simulink model "Replay_sim"  (Simulink 7.8)
settings: Solver=FixedStepDiscrete  StartTime=0.0  StopTime=valid_range_time(end)  FixedStep=T_step  RelTol=1e-3
InitFcn:
  | Replay_sim_init
values from neighbouring files (symbols this model uses):
  InitialPoint = 0    [boat_constants.m]    (also in l2plus.m)
  IPStar = 0    [boat_constants.m]    (also in l2plus.m)
  lla_ltp_gain = [r * (pi / 180 / 1e7); v * cos(ref_lla(1)) * (pi / 180 / 1e7); 1e-6]    [common.m]
  MaxDwnPthStar = 1    [boat_constants.m]    (also in l2plus.m)
  switchDistance = 4    [boat_constants.m]    (also in l2plus.m)
  T_step = 0.01    [boat_constants.m]    (also in common.m)
  tanIntercept = tan( 45*pi/180 )    [boat_constants.m]    (also in l2plus.m)
  TStar = single(4.5)    [boat_constants.m]    (also in l2plus.m = single(2))
  Turn2Track = 0    [boat_constants.m]    (also in l2plus.m)
  wheelbase = 3.27    [boat_constants.m]
undefined symbols (not defined in the file or in its folder): cogDotDerivativeDelay, DiscIntNeverNeededParam, gpsOrigin, KPsiDot
settings Model: Creator=Bryant  LastModifiedBy=Bryant
settings OptimizationCC: LifeSpan=30

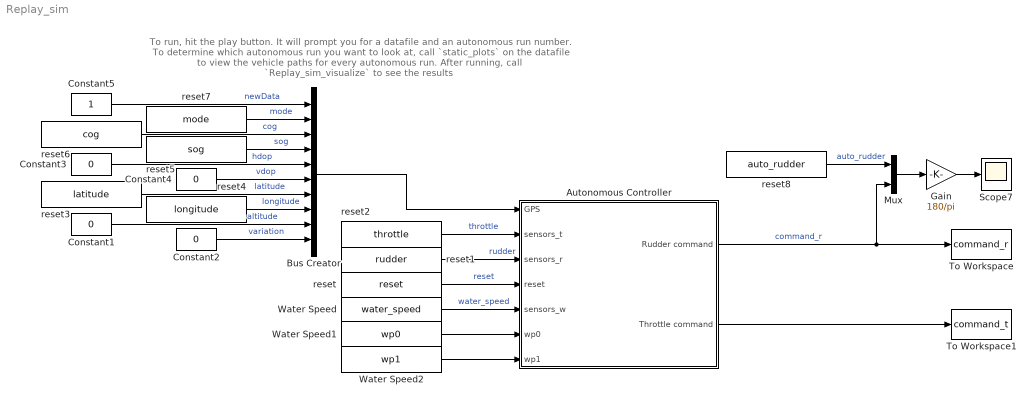
== system Replay_sim ==
  note: To run, hit the play button. It will prompt you for a datafile and an autonomous run number.
      |
      | To determine which autonomous run you want to look at, call `static_plots` on the datafile to
      | view the vehicle paths for every autonomous run.
      |
      | After running, call `Replay_sim_visualize` to see the results
  Autonomous Controller : Subsystem  Priority=1
  Bus Creator : BusCreator  Inputs=10  OutDataTypeStr=Bus: GpsData
  Constant1 : Constant  Value=0  OutDataTypeStr=int32
  Constant2 : Constant  Value=0  OutDataTypeStr=single
  Constant3 : Constant  Value=0  OutDataTypeStr=int16
  Constant4 : Constant  Value=0  OutDataTypeStr=int16
  Constant5 : Constant  OutDataTypeStr=boolean
  Gain : Gain  Gain=180/pi
  Mux : Mux  Inputs=2
  Scope7 : Scope
      settings: SaveName=ScopeData7
  To Workspace : ToWorkspace  VariableName=command_r  SampleTime=-1  SaveFormat=Structure With Time
  To Workspace1 : ToWorkspace  VariableName=command_t  SampleTime=-1  SaveFormat=Structure With Time
  Water Speed : FromWorkspace  VariableName=water_speed  SampleTime=T_step  Interpolate=off  OutputAfterFinalValue=Holding final value
  Water Speed1 : FromWorkspace  VariableName=wp0  SampleTime=T_step  Interpolate=off  OutputAfterFinalValue=Holding final value
  Water Speed2 : FromWorkspace  VariableName=wp1  SampleTime=T_step  Interpolate=off  OutputAfterFinalValue=Holding final value
  reset : FromWorkspace  VariableName=reset  SampleTime=T_step  Interpolate=off  OutputAfterFinalValue=Holding final value
  reset1 : FromWorkspace  VariableName=rudder  SampleTime=T_step  Interpolate=off  OutputAfterFinalValue=Holding final value
  reset2 : FromWorkspace  VariableName=throttle  SampleTime=T_step  Interpolate=off  OutputAfterFinalValue=Holding final value
  reset3 : FromWorkspace  VariableName=latitude  SampleTime=T_step  Interpolate=off  OutputAfterFinalValue=Holding final value
  reset4 : FromWorkspace  VariableName=longitude  SampleTime=T_step  Interpolate=off  OutputAfterFinalValue=Holding final value
  reset5 : FromWorkspace  VariableName=sog  SampleTime=T_step  Interpolate=off  OutputAfterFinalValue=Holding final value
  reset6 : FromWorkspace  VariableName=cog  SampleTime=T_step  Interpolate=off  OutputAfterFinalValue=Holding final value
  reset7 : FromWorkspace  VariableName=mode  SampleTime=T_step  Interpolate=off  OutputAfterFinalValue=Holding final value
  reset8 : FromWorkspace  VariableName=auto_rudder  SampleTime=T_step  Interpolate=off  OutputAfterFinalValue=Holding final value
  wires:
  Water Speed/1 -> Autonomous Controller/5(sensors_w)  "water_speed"
  Autonomous Controller/2(Throttle command) -> To Workspace1/1
  Autonomous Controller/1(Rudder command) -> To Workspace/1, Mux/2  "command_r"
  reset/1 -> Autonomous Controller/4(reset)  "reset"
  reset1/1 -> Autonomous Controller/3(sensors_r)  "rudder"
  reset2/1 -> Autonomous Controller/2(sensors_t)  "throttle"
  reset3/1 -> Bus Creator/7  "latitude"
  Bus Creator/1 -> Autonomous Controller/1(GPS)
  reset4/1 -> Bus Creator/8  "longitude"
  Constant2/1 -> Bus Creator/10  "variation"
  Constant1/1 -> Bus Creator/9  "altitude"
  Constant4/1 -> Bus Creator/6  "vdop"
  Constant3/1 -> Bus Creator/5  "hdop"
  reset5/1 -> Bus Creator/4  "sog"
  reset6/1 -> Bus Creator/3  "cog"
  reset7/1 -> Bus Creator/2  "mode"
  Constant5/1 -> Bus Creator/1  "newData"
  Mux/1 -> Gain/1
  reset8/1 -> Mux/1  "auto_rudder"
  Water Speed2/1 -> Autonomous Controller/7(wp1)
  Water Speed1/1 -> Autonomous Controller/6(wp0)
  Gain/1 -> Scope7/1

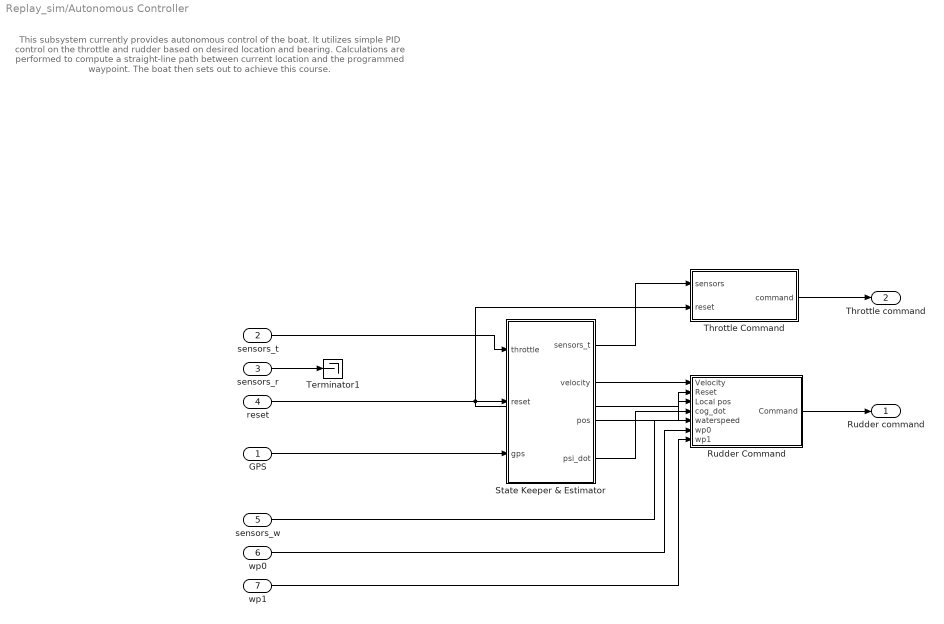
== system Replay_sim/Autonomous Controller ==
  note: This subsystem currently provides autonomous control of the boat. It utilizes simple PID control
      | on the throttle and rudder based on desired location and bearing. Calculations are performed
      | to compute a straight-line path between current location and the programmed waypoint. The
      | boat then sets out to achieve this course.
  GPS : Inport
  sensors_t : Inport  Port=2
  sensors_r : Inport  Port=3
  reset : Inport  Port=4
  sensors_w : Inport  Port=5
  wp0 : Inport  Port=6
  wp1 : Inport  Port=7
  Rudder Command : Subsystem
  State Keeper & Estimator : Subsystem
  Terminator1 : Terminator
  Throttle Command : Subsystem
  Rudder command : Outport
  Throttle command : Outport  Port=2
  wires:
  reset/1 -> Rudder Command/2(Reset), Throttle Command/2(reset), State Keeper & Estimator/2(reset)
  State Keeper & Estimator/3(pos) -> Rudder Command/3(Local pos)
  State Keeper & Estimator/1(sensors_t) -> Throttle Command/1(sensors)
  State Keeper & Estimator/2(velocity) -> Rudder Command/1(Velocity)
  GPS/1 -> State Keeper & Estimator/3(gps)
  Throttle Command/1(command) -> Throttle command/1
  Rudder Command/1(Command) -> Rudder command/1
  sensors_r/1 -> Terminator1/1
  sensors_t/1 -> State Keeper & Estimator/1(throttle)
  State Keeper & Estimator/4(psi_dot) -> Rudder Command/4(cog_dot)
  sensors_w/1 -> Rudder Command/5(waterspeed)
  wp0/1 -> Rudder Command/6(wp0)
  wp1/1 -> Rudder Command/7(wp1)

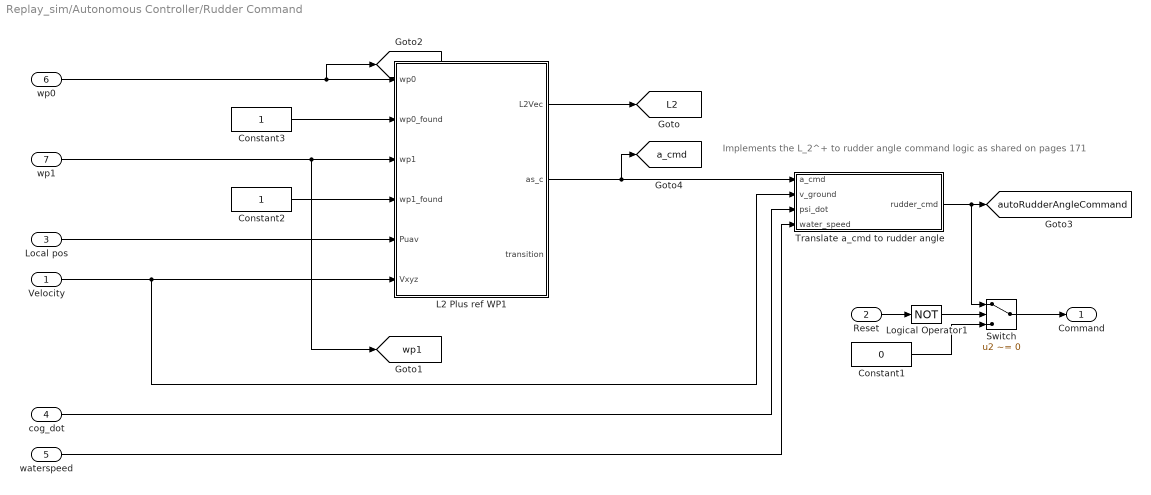
== system Replay_sim/Autonomous Controller/Rudder Command ==
  note: Implements the L_2^+ to rudder angle command logic as shared on pages 171
  Velocity : Inport
  Reset : Inport  Port=2
  Local pos : Inport  Port=3
  cog_dot : Inport  Port=4
  waterspeed : Inport  Port=5
  wp0 : Inport  Port=6
  wp1 : Inport  Port=7
  Constant1 : Constant  Value=0  OutDataTypeStr=single
  Constant2 : Constant  OutDataTypeStr=boolean
  Constant3 : Constant  OutDataTypeStr=boolean
  L2 Plus ref WP1 : MATLAB Function  TreatAsAtomicUnit=on
  Logical Operator1 : Logic  Operator=NOT  Inputs=1  AllPortsSameDT=off  OutDataTypeStr=boolean
  Switch : Switch  Criteria=u2 ~= 0
  Translate a_cmd to rudder angle : Subsystem
  Command : Outport
  tag scope: L2=global, a_cmd=global, autoRudderAngleCommand=global, wp0=global, wp1=global
  wires:
  wp0/1 -> L2 Plus ref WP1/1(wp0), [wp0]
  wp1/1 -> L2 Plus ref WP1/3(wp1), [wp1]
  Local pos/1 -> L2 Plus ref WP1/5(Puav)
  Velocity/1 -> L2 Plus ref WP1/6(Vxyz), Translate a_cmd to rudder angle/2(v_ground)
  L2 Plus ref WP1/1(L2Vec) -> [L2]
  Translate a_cmd to rudder angle/1(rudder_cmd) -> [autoRudderAngleCommand], Switch/1
  Reset/1 -> Logical Operator1/1
  Constant1/1 -> Switch/3
  Switch/1 -> Command/1
  Logical Operator1/1 -> Switch/2
  L2 Plus ref WP1/2(as_c) -> [a_cmd], Translate a_cmd to rudder angle/1(a_cmd)
  cog_dot/1 -> Translate a_cmd to rudder angle/3(psi_dot)
  waterspeed/1 -> Translate a_cmd to rudder angle/4(water_speed)
  Constant3/1 -> L2 Plus ref WP1/2(wp0_found)
  Constant2/1 -> L2 Plus ref WP1/4(wp1_found)

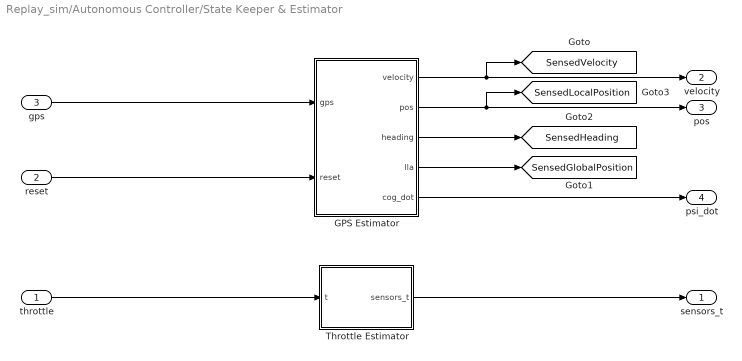
== system Replay_sim/Autonomous Controller/State Keeper & Estimator ==
  throttle : Inport
  reset : Inport  Port=2
  gps : Inport  Port=3
  GPS Estimator : Subsystem
  Throttle Estimator : Subsystem
  sensors_t : Outport
  velocity : Outport  Port=2
  pos : Outport  Port=3
  psi_dot : Outport  Port=4
  tag scope: SensedGlobalPosition=global, SensedHeading=global, SensedLocalPosition=global, SensedVelocity=global
  wires:
  Throttle Estimator/1(sensors_t) -> sensors_t/1
  GPS Estimator/4(lla) -> [SensedGlobalPosition]
  GPS Estimator/3(heading) -> [SensedHeading]
  GPS Estimator/2(pos) -> [SensedLocalPosition], pos/1
  gps/1 -> GPS Estimator/1(gps)
  GPS Estimator/1(velocity) -> [SensedVelocity], velocity/1
  reset/1 -> GPS Estimator/2(reset)
  throttle/1 -> Throttle Estimator/1(t)
  GPS Estimator/5(cog_dot) -> psi_dot/1

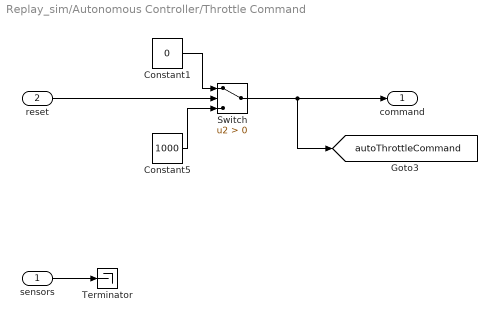
== system Replay_sim/Autonomous Controller/Throttle Command ==
  sensors : Inport
  reset : Inport  Port=2
  Constant1 : Constant  Value=0  OutDataTypeStr=int16
  Constant5 : Constant  Value=1000  OutDataTypeStr=int16
  Switch : Switch  Criteria=u2 > Threshold
  Terminator : Terminator
  command : Outport
  tag scope: autoThrottleCommand=global
  wires:
  Constant5/1 -> Switch/3
  Constant1/1 -> Switch/1
  reset/1 -> Switch/2
  sensors/1 -> Terminator/1
  Switch/1 -> [autoThrottleCommand], command/1

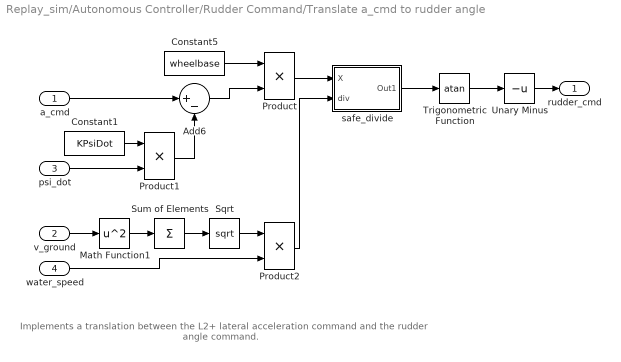
== system Replay_sim/Autonomous Controller/Rudder Command/Translate a_cmd to rudder angle ==
  note: Implements a translation between the L2+ lateral acceleration command
      | and the rudder angle command.
  a_cmd : Inport
  v_ground : Inport  Port=2
  psi_dot : Inport  Port=3
  water_speed : Inport  Port=4
  Add6 : Sum  Inputs=|+-
  Constant1 : Constant  Value=KPsiDot
  Constant5 : Constant  Value=wheelbase
  Math Function1 : Math  Operator=square  SaturateOnIntegerOverflow=on
  Product : Product  Inputs=**  RndMeth=Zero
  Product1 : Product  Inputs=**  RndMeth=Zero
  Product2 : Product  Inputs=**  RndMeth=Zero
  Sqrt : Sqrt  SaturateOnIntegerOverflow=on
  Sum of Elements : Sum  Inputs=+
  Trigonometric Function : Trigonometry  Operator=atan
  Unary Minus : UnaryMinus
  safe_divide : Subsystem  TreatAsAtomicUnit=on
      settings: RTWFcnNameOpts=Use subsystem name  RTWFileNameOpts=Use function name
  rudder_cmd : Outport
  wires:
  Constant5/1 -> Product/1
  Product/1 -> safe_divide/1(X)
  Trigonometric Function/1 -> Unary Minus/1
  Math Function1/1 -> Sum of Elements/1
  Sum of Elements/1 -> Sqrt/1
  safe_divide/1(Out1) -> Trigonometric Function/1
  Add6/1 -> Product/2
  Product1/1 -> Add6/2
  v_ground/1 -> Math Function1/1
  Unary Minus/1 -> rudder_cmd/1
  a_cmd/1 -> Add6/1
  psi_dot/1 -> Product1/2
  Constant1/1 -> Product1/1
  Sqrt/1 -> Product2/1
  Product2/1 -> safe_divide/2(div)
  water_speed/1 -> Product2/2

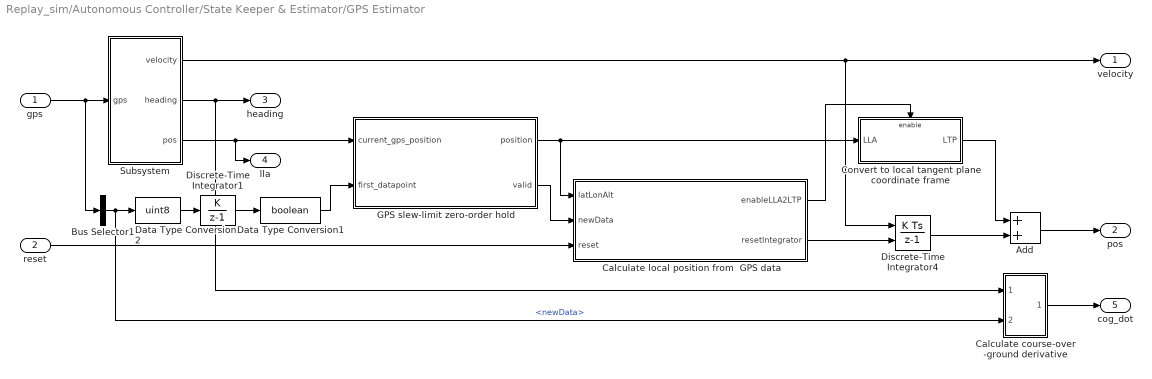
== system Replay_sim/Autonomous Controller/State Keeper & Estimator/GPS Estimator ==
  gps : Inport
  reset : Inport  Port=2
  Add : Sum
  Bus Selector1 : BusSelector  OutputSignals=newData
  Calculate course-over-ground derivative : Subsystem
  Calculate local position from  GPS data : MATLAB Function  TreatAsAtomicUnit=on
  Convert to local tangent plane coordinate frame : Subsystem  TreatAsAtomicUnit=on  RTWFcnName=lla2ltp
      settings: RTWFcnNameOpts=User specified
  Data Type Conversion1 : DataTypeConversion  OutDataTypeStr=boolean
  Data Type Conversion2 : DataTypeConversion  OutDataTypeStr=uint8
  Discrete-Time Integrator1 : DiscreteIntegrator  IntegratorMethod=Accumulation: Forward Euler  SampleTime=-1  OutDataTypeStr=uint8  RndMeth=Simplest  LimitOutput=on  UpperSaturationLimit=1  LowerSaturationLimit=0  ICPrevOutput=DiscIntNeverNeededParam  ICPrevScaledInput=DiscIntNeverNeededParam
  Discrete-Time Integrator4 : DiscreteIntegrator  ExternalReset=level  SampleTime=-1  ICPrevOutput=DiscIntNeverNeededParam  ICPrevScaledInput=DiscIntNeverNeededParam
  GPS slew-limit zero-order hold : MATLAB Function  TreatAsAtomicUnit=on
  Subsystem : Subsystem
  velocity : Outport
  pos : Outport  Port=2
  heading : Outport  Port=3
  lla : Outport  Port=4
  cog_dot : Outport  Port=5
  wires:
  Subsystem/1(velocity) -> Discrete-Time Integrator4/1, velocity/1
  Calculate local position from  GPS data/2(resetIntegrator) -> Discrete-Time Integrator4/2
  Add/1 -> pos/1
  Discrete-Time Integrator4/1 -> Add/2
  Subsystem/3(pos) -> lla/1, GPS slew-limit zero-order hold/1(current_gps_position)
  gps/1 -> Bus Selector1/1, Subsystem/1(gps)
  Subsystem/2(heading) -> heading/1, Calculate course-over-ground derivative/1(cog)
  reset/1 -> Calculate local position from  GPS data/3(reset)
  Convert to local tangent plane coordinate frame/1(LTP) -> Add/1
  Calculate local position from  GPS data/1(enableLLA2LTP) -> Convert to local tangent plane coordinate frame/Enable
  Discrete-Time Integrator1/1 -> Data Type Conversion1/1
  GPS slew-limit zero-order hold/1(position) -> Calculate local position from  GPS data/1(latLonAlt), Convert to local tangent plane coordinate frame/1(LLA)
  GPS slew-limit zero-order hold/2(valid) -> Calculate local position from  GPS data/2(newData)
  Bus Selector1/1 -> Calculate course-over-ground derivative/2(new), Data Type Conversion2/1  "<newData>"
  Data Type Conversion1/1 -> GPS slew-limit zero-order hold/2(first_datapoint)
  Data Type Conversion2/1 -> Discrete-Time Integrator1/1
  Calculate course-over-ground derivative/1(cog_dot) -> cog_dot/1

== system Replay_sim/Autonomous Controller/State Keeper & Estimator/Throttle Estimator ==
  t : Inport
  sensors_t : Outport
  wires:
  t/1 -> sensors_t/1

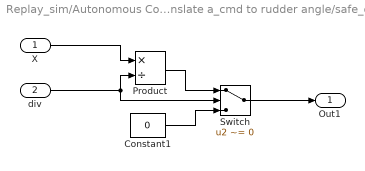
== system Replay_sim/Autonomous Controller/Rudder Command/Translate a_cmd to rudder angle/safe_divide ==
  X : Inport
  div : Inport  Port=2
  Constant1 : Constant  Value=0  OutDataTypeStr=Inherit: Inherit via back propagation
  Product : Product  Inputs=*/  RndMeth=Zero
  Switch : Switch  Criteria=u2 ~= 0
  Out1 : Outport
  wires:
  X/1 -> Product/1
  div/1 -> Product/2, Switch/2
  Product/1 -> Switch/1
  Constant1/1 -> Switch/3
  Switch/1 -> Out1/1

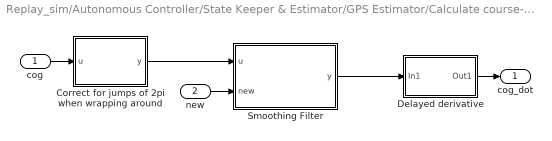
== system Replay_sim/Autonomous Controller/State Keeper & Estimator/GPS Estimator/Calculate course-over-ground derivative ==
  cog : Inport
  new : Inport  Port=2
  Correct for jumps of 2pi when wrapping around : MATLAB Function  TreatAsAtomicUnit=on
  Delayed derivative : Subsystem  mask{delay=cogDotDerivativeDelay, Ts=.01}
      mask prompts: delay "Delay (s)"; Ts "Sample time"
      mask Display: text(0.5,0.5,'Der');
  Smoothing Filter : Subsystem  mask{gain=0.5, limit=8, Ts=.01, freq=.3}
      mask prompts: Ts "Sample time"; freq "Lowpass frequency"
  cog_dot : Outport
  wires:
  Smoothing Filter/1(y) -> Delayed derivative/1(In1)
  Correct for jumps of 2pi when wrapping around/1(y) -> Smoothing Filter/1(u)
  cog/1 -> Correct for jumps of 2pi when wrapping around/1(u)
  Delayed derivative/1(Out1) -> cog_dot/1
  new/1 -> Smoothing Filter/2(new)

== system Replay_sim/Autonomous Controller/State Keeper & Estimator/GPS Estimator/Convert to local tangent plane coordinate frame ==
  LLA : Inport
  Enable : EnablePort
  LLA2LTP : Subsystem  TreatAsAtomicUnit=on  RTWFcnName=lla2ltp
      settings: RTWFcnNameOpts=User specified
  LTP : Outport  OutDataTypeStr=single  InitialOutput=[0, 0, 0]
  wires:
  LLA/1 -> LLA2LTP/1(LLA)
  LLA2LTP/1(LTP) -> LTP/1

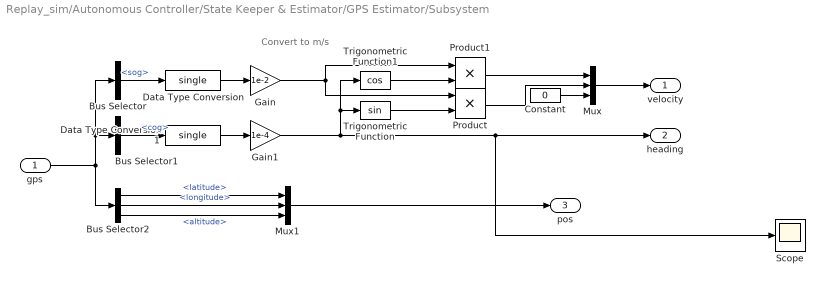
== system Replay_sim/Autonomous Controller/State Keeper & Estimator/GPS Estimator/Subsystem ==
  note: Convert to m/s
  gps : Inport
  Bus Selector : BusSelector  OutputSignals=sog
  Bus Selector1 : BusSelector  OutputSignals=cog
  Bus Selector2 : BusSelector  OutputSignals=latitude,longitude,altitude
  Constant : Constant  Value=0  OutDataTypeStr=single
  Data Type Conversion : DataTypeConversion  OutDataTypeStr=single  RndMeth=Simplest
  Data Type Conversion1 : DataTypeConversion  OutDataTypeStr=single  RndMeth=Simplest
  Gain : Gain  Gain=1e-2
  Gain1 : Gain  Gain=1e-4
  Mux : Mux  Inputs=3
  Mux1 : Mux  Inputs=3
  Product : Product  OutDataTypeStr=single  RndMeth=Zero
  Product1 : Product  OutDataTypeStr=single  RndMeth=Zero
  Scope : Scope
      settings: YMin=1.6  YMax=1.825
  Trigonometric Function : Trigonometry
  Trigonometric Function1 : Trigonometry  Operator=cos
  velocity : Outport
  heading : Outport  Port=2
  pos : Outport  Port=3
  wires:
  gps/1 -> Bus Selector/1, Bus Selector1/1, Bus Selector2/1
  Bus Selector1/1 -> Data Type Conversion1/1  "<cog>"
  Trigonometric Function/1 -> Product/2
  Trigonometric Function1/1 -> Product1/2
  Product1/1 -> Mux/1
  Product/1 -> Mux/2
  Constant/1 -> Mux/3
  Mux/1 -> velocity/1
  Bus Selector/1 -> Data Type Conversion/1  "<sog>"
  Bus Selector2/2 -> Mux1/2  "<longitude>"
  Bus Selector2/3 -> Mux1/3  "<altitude>"
  Mux1/1 -> pos/1
  Bus Selector2/1 -> Mux1/1  "<latitude>"
  Data Type Conversion/1 -> Gain/1
  Data Type Conversion1/1 -> Gain1/1
  Gain/1 -> Product1/1, Product/1
  Gain1/1 -> Trigonometric Function/1, Trigonometric Function1/1, heading/1, Scope/1

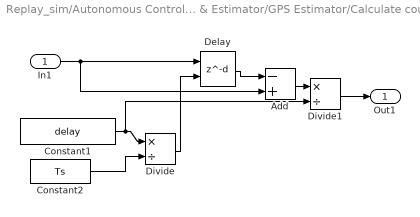
== system Replay_sim/Autonomous Controller/State Keeper & Estimator/GPS Estimator/Calculate course-over-ground derivative/Delayed derivative ==
  In1 : Inport
  Add : Sum  Inputs=-+
  Constant1 : Constant  Value=delay  OutDataTypeStr=single  SampleTime=.01
  Constant2 : Constant  Value=Ts  OutDataTypeStr=single
  Delay : Delay  DelayLengthSource=Input port  DelayLength=delay/Ts  DelayLengthUpperLimit=1000  DiagnosticForOutOfRangeDelayLength=Error  RemoveProtectionDelayLength=on  UseCircularBuffer=on  SampleTime=.01
      settings: InputPortMap=u0,p1
  Divide : Product  Inputs=*/
  Divide1 : Product  Inputs=*/
  Out1 : Outport
  wires:
  Delay/1 -> Add/1
  Add/1 -> Divide1/1
  In1/1 -> Delay/1, Add/2
  Divide1/1 -> Out1/1
  Divide/1 -> Delay/2
  Constant1/1 -> Divide1/2, Divide/1
  Constant2/1 -> Divide/2

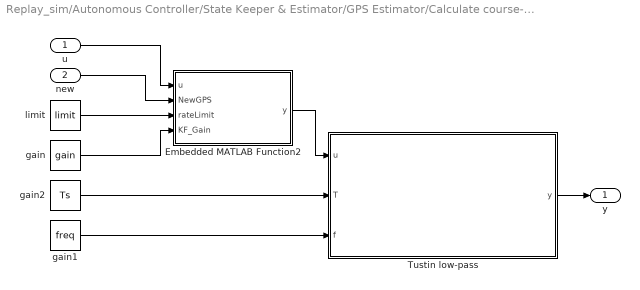
== system Replay_sim/Autonomous Controller/State Keeper & Estimator/GPS Estimator/Calculate course-over-ground derivative/Smoothing Filter ==
  u : Inport  OutDataTypeStr=single
  new : Inport  Port=2  OutDataTypeStr=boolean
  Embedded MATLAB Function2 : MATLAB Function  TreatAsAtomicUnit=on
  Tustin low-pass : MATLAB Function  TreatAsAtomicUnit=on
  gain : Constant  Value=gain  OutDataTypeStr=Inherit: Inherit via back propagation
  gain1 : Constant  Value=freq  OutDataTypeStr=Inherit: Inherit via back propagation
  gain2 : Constant  Value=Ts  OutDataTypeStr=Inherit: Inherit via back propagation
  limit : Constant  Value=limit  OutDataTypeStr=Inherit: Inherit via back propagation
  y : Outport  OutputWhenDisabled=reset  InitialOutput=0
  wires:
  Embedded MATLAB Function2/1(y) -> Tustin low-pass/1(u)
  u/1 -> Embedded MATLAB Function2/1(u)
  new/1 -> Embedded MATLAB Function2/2(NewGPS)
  limit/1 -> Embedded MATLAB Function2/3(rateLimit)
  gain/1 -> Embedded MATLAB Function2/4(KF_Gain)
  Tustin low-pass/1(y) -> y/1
  gain2/1 -> Tustin low-pass/2(T)
  gain1/1 -> Tustin low-pass/3(f)

== system Replay_sim/Autonomous Controller/State Keeper & Estimator/GPS Estimator/Convert to local tangent plane coordinate frame/LLA2LTP ==
  LLA : Inport
  Add : Sum  Inputs=+-  OutDataTypeStr=double  RndMeth=Simplest
  Constant : Constant  Value=gpsOrigin  OutDataTypeStr=int32
  Constant1 : Constant  Value=lla_ltp_gain  OutDataTypeStr=double
  Product : Product  OutDataTypeStr=single  RndMeth=Simplest  LockScale=on
  LTP : Outport  OutDataTypeStr=single  InitialOutput=[0, 0, 0]
  wires:
  Add/1 -> Product/1
  Constant1/1 -> Product/2
  Product/1 -> LTP/1
  Constant/1 -> Add/2
  LLA/1 -> Add/1

== matlab function Autonomous Controller/State Keeper & Estimator/GPS Estimator/Calculate course-over-ground derivative/Correct for jumps of 2pi when wrapping around ==
  data: u input single size=1; y output single size=1
function y = jumpfix(u)
%#codegen

% Initialize values
persistent lastU offset firstDatum;
if isempty(lastU)
    lastU = single(0);
    offset = single(0);
    firstDatum = true;
end

% Latch the first input so we don't have a huge step going from 0 to the
% first input.
if firstDatum
    lastU = u;
    firstDatum = false;
end

% Wrap the values depending on the 
if u - lastU > pi
    offset = offset - 2*pi;
elseif u -lastU < -pi
    offset = offset + 2*pi;
end

% And store the current data point for next time.
lastU = u;

% Output the corrected value
y = u + offset;

== matlab function Autonomous Controller/State Keeper & Estimator/GPS Estimator/Calculate local position from GPS data ==
  data: enableLLA2LTP output boolean size=1; latLonAlt input int32 size=3; newData input boolean size=1; reset input boolean size=1; resetIntegrator output boolean size=1
function [enableLLA2LTP, resetIntegrator]  = estimateGPS(latLonAlt, newData, reset)
%#codegen

% This function watches an incoming stream of GPS data and waits for 5
% valid LLA values before it enables LLA to LTP conversion. It also watches
% for updates to a GPS stream in order to reset a velocity integrator for
% position estimation.

% INPUTS:
% latLonAlt - the latitude, longitude, and altitude of the vehicle from GPS
% in radians/meters.
% newData - A boolean signal specifying whether latLonAlt holds new data
% reset - A global reset boolean trigger.

% OUTPUTS:
% enableLLA2LTP - A boolean specifying whether LLA to LTP conversion should
% occur. The only reason it shouldn't is if the GPS hasn't latched valid
% positions yet.
% resetIntegrator - Indicates that the velocity integrator, which is
% calculating position in between GPS fixes, should be reset.

persistent newDataCounter;

% Reset everything on first startup or when a global reset is triggered
if isempty(newDataCounter) || reset
    newDataCounter = uint8(0);
end

% Pass through the global reset to the velocity integrator
if reset
    resetIntegrator = true;
else
    resetIntegrator = false;
end

% Wait for 5 valid GPS inputs before outputting the current position.
% This allows the GPS to stabilize.
if newDataCounter < 5
    if newData && latLonAlt(1) ~= 0 && latLonAlt(2) ~= 0
        newDataCounter = newDataCounter + 1;
    end
    enableLLA2LTP = false;
else
    % Reset the integrator if new data has been received for this timestep
    % as we have a "truth" position now.
    if newData
        resetIntegrator = true;
    end
    enableLLA2LTP = true;
end

== matlab function Autonomous Controller/State Keeper & Estimator/GPS Estimator/GPS slew-limit zero-order hold ==
  data: position output int32 size=3; current_gps_position input int32 size=3; first_datapoint input boolean size=1; gps_leap_rate_limit parameter int32 size=1; valid output boolean size=1
function [position, valid] = limit_gps_rate(current_gps_position, first_datapoint, gps_leap_rate_limit)
%% This function follows a GPS position 2-tuple of lat/lon values (stored as int32s as 1e-7 degrees).
%#codegen

% Store the last GPS location, used for derivative calculations
persistent last_gps_position last_timestep current_timestep
if isempty(last_gps_position) || first_datapoint
    last_gps_position = current_gps_position;
    current_timestep = int32(0);
    last_timestep = current_timestep;
end

% If the slew limit was exceeded for either the latitude or longitude, only
% output the last timestep. We ignore the altitude completely.
if (current_gps_position(1) - last_gps_position(1)) / (current_timestep - last_timestep) > gps_leap_rate_limit ...
    || (current_gps_position(2) - last_gps_position(2)) / (current_timestep - last_timestep) > gps_leap_rate_limit
    position = last_gps_position;
    valid = false;
else
    % Update last timesteps data for future calculations.
    last_gps_position = current_gps_position;
    last_timestep = current_timestep;
    
    % We can output the current position as it's within the slew limit.
    position = current_gps_position;
    valid = true;
end

% Increment the current timestep handling wrap-arounds nicely. This WILL
% NOT handle situations were the time between valid GPS position updates is
% greater than INT32_MAX, but I can live with that.
if current_timestep == intmax('int32')
    current_timestep = current_timestep - last_timestep;
    last_timestep = int32(0);
else
    current_timestep = current_timestep + int32(1);
end

== matlab function Autonomous Controller/Rudder Command/L2 Plus ref WP1 ==
  data: wp0 input single size=3; wp0_found input boolean size=1; wp1 input single size=3; wp1_found input boolean size=1; L2Vec output single size=3; Puav input single size=3; Vxyz input single size=3; switchDistance parameter double size=1; tanIntercept parameter double size=1; MaxDwnPthStar parameter double size=1; Turn2Track parameter double size=1; InitialPoint parameter double size=1; IPStar parameter double size=1; TStar parameter double size=1; as_c output single size=1; transition output boolean size=1
function [L2Vec, as_c, transition] = L2PlusWP1(wp0, wp0_found, wp1, wp1_found, Puav, Vxyz, switchDistance, ...
    tanIntercept, MaxDwnPthStar,Turn2Track,...
    InitialPoint, IPStar, TStar)
%==============================
%     computes bank angle command for following a straight line
%     by creating an aim point that may be more than L2 away 
%     from the UAV. The aim point is (usually) farther along the path 
%     toward wp1 than the UAV, and the intercept
%     angle is less than or equal to a specified value. This limits the intercept
%     angle even when the UAV is within L2 of the path.
%     See L2PlusWP1.m for details
%
%         INPUTS
%             wp0     Waypoint 0 position in North-East-Down meters
%             wp1     Waypoint 1 position in North-East-Down meters
%             Puav    Position of UAV in North-East-Down meters
%             Vxyz    Inertial velocity in North-East-Down meters
%
%         PARAMETERS
%             switchDistance distance from wp1 to switch to WP2
%             tanIntercept  tangent of intercept angle
%             MaxDwnPthStar L2 multiplier to determmine downpath aimpoint
%             Turn2Track    true to turn toward T1 instead of L2
%             InitialPoint  true if no line tracking at first--fly direct to some initial point
%             IPStar        L2 multiplier to determing distance of IP from first wp0
%             Tstar         was called L2Base, time constant of response
%             
%         OUTPUTS
%             L2Vec   L2 vector toward aim point
%             as_c    commanded lateral acceleration. Values of 99/-99
%                     indicate saturated maximum/minimum.
%             transition A boolean of whether to transition or not to the next waypoint

    persistent IPActive;  %true if flying toward IP
    persistent IP; % location of initial point

    persistent direction; % Keep track of the direction for patrol mode
    if isempty(direction)
        direction = int8(1);
    end
    
    Pwp1 = single(zeros(3,1));
    Pe_y = single(0);
    Dist2wp1 = single(0);
    MinDownPath = single(0);
    Dist2WPSwitch = single(0);
    L2DownPath = single(0);
    L2ToT = single(zeros(3,1));
    L2Vec = single(zeros(3,1));
    IP1 = single([0; 0;-999]); %signal for no IP
    as_c = single(0);
    transition = false;
    
    Pne = [Puav(1); Puav(2); 0]; %horizontal position
    Vne = [Vxyz(1); Vxyz(2); 0]; % horizontal velocity
    Groundspeed = norm(Vne);
    L2 = single(TStar*Groundspeed);
    
    % If neither waypoint is valid then don't do anything
    if ~wp0_found || ~wp1_found
        return;
    % Otherwise if the first two waypoints are next to each other (as is
    % common if the origin is the first waypoint and the boat latches that
    % as its start value) then transition to the next waypoint.
    elseif norm(wp1 - wp0) < switchDistance
        transition = true;
        return;
    end
    
    % Calculate N1 (right-hand orthogonal to T1) 
    % and T1 (unit vector pointing from wp0 to wp1)
    T1 = wp1 - wp0;
    T1 = T1/norm(T1);
    N1 = [-T1(2); T1(1); 0];
    
%     initialize the initial point
    if (isempty(IPActive))
        if (InitialPoint)
%             IP is set relative to the first "from" waypoint
            IPActive = -1;
            IP = [wp0(1); wp0(2); 0] - L2*IPStar*T1;
            
            if (norm(IP-Pne) < .001)
                IPActive = 0;
                IP = single([0; 0; -999]);
            end
        else
            IPActive = 0;
            IP = single([0; 0;-999]); %signal for no IP
        end
    end
    IP1 = IP;
    
    
    if (IPActive)
%         no line tracking, direct to IP
        L2Vec = L2*(IP - Pne)/norm(IP - Pne);
%         check to see if at the IP to terminate this mode
        if norm(IP - Pne) < .1*L2
            IPActive = 0;
        end
    else
         if (Pne(1) < 2)
             IP1 = IP1;
         end
%         IP not active, track WP lines
        Pwp1 = Pne - [wp1(1); wp1(2); 0]; % position of UAV relative to wp1
        Pe_y = single(Pwp1'*N1); % cross track error
        Dist2wp1 = -single(Pwp1'*T1); % distance to wp1

%         minimum down path distance for Aim Point intersection on T
%         is determined by the intercept angle but limited 
%         in case of very distant intecepts to MaxDwnPthStar*L2
        MinDownPath = single ( min( abs(Pe_y)/tanIntercept, MaxDwnPthStar*L2)); 
        Dist2WPSwitch = Dist2wp1 - switchDistance;
        if ( abs(Pe_y) > L2 )
    %             Make sure aimpoint is no closer to waypoint than calculated switch point.
            L2DownPath = MinDownPath;
        else
    %             within L2 of T and Dist2WPSwitch >= 0, but limit angle of L2 wrt T
            L2DownPath = (max(MinDownPath, (sqrt( L2^2 - Pe_y^2 ))));
        end
        
        if ( Dist2WPSwitch < 0 )
            transition = true;
        end
        
         % vector from Pwp1 to aim point on T1
         L2ToT = single(( Dist2wp1 - L2DownPath )*(-T1) - Pwp1);
         if (norm(L2ToT) < .001)
             L2Vec = L2*T1;
         else
            L2Vec = single(L2*( L2ToT/norm(L2ToT) )); % limit size to L2
         end
    %         L2Vec = L2ToT;
%         dummy statements
    end
    Zprod = single(Vxyz(1)*L2Vec(2) - Vxyz(2)*L2Vec(1)); %Z component of cross product
    
    % Now if the groundspeed of the vessel is zero, we make sure we don't
    % get a division-by-zero error and instead handle it gracefully.
    if Groundspeed > 0
        sinEta = single(Zprod/(Groundspeed*L2));
        as_c = single(2*Groundspeed^2/(L2)*sinEta);
    else
        sinEta = single(0.0);
        as_c = single(0.0);
    end

%         now override bank angle if heading in the wrong direction
    if ( Turn2Track && Dist2WPSwitch > 0 && ~IPActive ) 
%             turn to track not L2, gives min displacement from track
        if ( T1'*Vxyz < 0 )
            if ( Pe_y > 0 )
                as_c = single(99);
            else
                as_c = single(-99);
            end
        end
     else
%           turn toward L2, give min displacement toward wp0
        if ( L2Vec'*Vxyz < 0 )
            if ( sinEta < 0 )
                as_c = single(-99);
            else
                as_c = single(99);
            end
        end
    end
end

== matlab function Autonomous Controller/State Keeper & Estimator/GPS Estimator/Calculate course-over-ground derivative/Smoothing Filter/Embedded MATLAB Function2 ==
  data: u input single size=1; y output single size=1; NewGPS input boolean size=1; Ts parameter single size=1; rateLimit input single; KF_Gain input single
function y = RateAid(u,NewGPS,Ts, rateLimit,KF_Gain)
% This function does a smoothing of the differences of input u
% to use as a rate estimate of the output until the next sample
% That output estimate is smoothed with the new measurement
% In other words, a heuristic Kalman Filter
% 
% INPUTS
%     u               signal to be filtered
%     NewGPS          pulse indicating a new GPS reading is availble
%     apSampleTime    sample time of the system
%     rateLimit       used to discard outliers
%     KF_Gain         Kalman gain for the filter (valid values are between
%                     0 and 1.0
% OUTPUTS
%     y        velocity estimate between updates. It is a sawtooth pattern, so
%             this routine is followed by a low pass filter
             
             
persistent TimeSinceLast;
persistent rate;
persistent rateHat;
persistent yHat;
persistent firstGPS;
persistent LastU;

if (isempty(LastU))
    LastU = single(0.);
    TimeSinceLast = single(Ts);
    rate = single(0);
    rateHat = single(0);
    yHat = single(0);
    firstGPS= single(1);
end

yHat = yHat + rateHat*Ts;
if (NewGPS && TimeSinceLast > 3*Ts) %needed for long GPS pulse
    if firstGPS == 1
%         initialize to first input
        yHat = u;
        y = u;
        firstGPS = single(0);
        return;
    end
    rateOld = rate;
    rate = single((u - LastU)/TimeSinceLast);
%     return with no change if outside accel limit
    if ( rate < -rateLimit || rate > rateLimit )
        rate = single(0);
        y = yHat; %no change to yHat
        return;
    end
%     rateHat = rateHat + .9*(rate - rateHat); %first order filter
    rateHat = .7*rate + .3*rateOld; %FIR filter
    TimeSinceLast = single(0);
    LastU = u;
    yHat = yHat +KF_Gain*( u - yHat ); 
end
y = yHat;
TimeSinceLast = TimeSinceLast + Ts;

== matlab function Autonomous Controller/State Keeper & Estimator/GPS Estimator/Calculate course-over-ground derivative/Smoothing Filter/Tustin low-pass ==
  data: u input double; y output single; T input double; f input double
function y = fcn(u,T,f)
% This block supports an embeddable subset of the MATLAB language.
% See the help menu for details. 

persistent a
persistent b
persistent y_km1
persistent u_km1
if isempty(a)
    %tf = [T*omega/(2+T*omega) T*omega/(2+T*omega)],[1 (T*omega-2)/(T*omega+2)]
    %tf = [a a],[1 -b]
    omega = 2*pi*f;
    a=T*omega/(2+T*omega);
    b=-(T*omega-2)/(T*omega+2);
    y_km1=u;
    u_km1=u;
end

y = single(a*(u+u_km1)+b*y_km1);
y_km1=y;
u_km1=u;
